simulink model "HDVPSG_DelayComp_NewRef_RealDrop_case1"  (R2019b)
settings: Solver=FixedStepDiscrete  StartTime=0.0  StopTime=28  FixedStep=UT.Ts_Veh  RelTol=1e-3
PostLoadFcn:
  | if any(exist('dsrtsu_mdlpostloadfcn', 'file') ~= 0), dsrtsu_mdlpostloadfcn('Execute', bdroot); end
InitFcn:
  | , if any(exist('dsmpb_private', 'file') ~= 0), dsmpb_private('dsmpb_mdlclblib', 'Init', bdroot); end,
values from neighbouring files (symbols this model uses):
  BETA_HDV_Leader = 50    [HDVPSG_DelayComp_NewRef_RealDrop_script_case1.m]
  BETA_PSG_Follower = 150    [HDVPSG_DelayComp_NewRef_RealDrop_script_case1.m]
  CtrlZone_Length = 250    [HDVPSG_DelayComp_NewRef_RealDrop_script_case1.m]
  DELTA_D_MIN = 5    [HDVPSG_DelayComp_NewRef_RealDrop_script_case1.m]
  DELTA_DR_MG_TCC = 15    [HDVPSG_DelayComp_NewRef_RealDrop_script_case1.m]
  HDV_AMAX = 1.3    [HDVPSG_DelayComp_NewRef_RealDrop_script_case1.m]
  HDV_AMIN = -2.5    [HDVPSG_DelayComp_NewRef_RealDrop_script_case1.m]
  HDV_first_v0 = 13    [HDVPSG_DelayComp_NewRef_RealDrop_script_case1.m]
  HDV_HighMu_D = 9    [HDVPSG_DelayComp_NewRef_RealDrop_script_case1.m]
  HDV_HighMu_I = 27    [HDVPSG_DelayComp_NewRef_RealDrop_script_case1.m]
  HDV_HighMu_P = 27    [HDVPSG_DelayComp_NewRef_RealDrop_script_case1.m]
  HDV_HighMu_TRFC = 0.7    [HDVPSG_DelayComp_NewRef_RealDrop_script_case1.m]
  HDV_last_v0 = 13    [HDVPSG_DelayComp_NewRef_RealDrop_script_case1.m]
  HDV_LowMu_D = 6    [HDVPSG_DelayComp_NewRef_RealDrop_script_case1.m]
  HDV_LowMu_I = 8    [HDVPSG_DelayComp_NewRef_RealDrop_script_case1.m]
  HDV_LowMu_P = 12    [HDVPSG_DelayComp_NewRef_RealDrop_script_case1.m]
  HDV_LowMu_TRFC = 0.6    [HDVPSG_DelayComp_NewRef_RealDrop_script_case1.m]
  Np_MPC = 20    [HDVPSG_DelayComp_NewRef_RealDrop_script_case1.m]
  PSG_AMAX = 3.2    [HDVPSG_DelayComp_NewRef_RealDrop_script_case1.m]
  PSG_AMIN = -6    [HDVPSG_DelayComp_NewRef_RealDrop_script_case1.m]
  PSG_end_v0 = 13    [HDVPSG_DelayComp_NewRef_RealDrop_script_case1.m]
  PSG_first_v0 = 13    [HDVPSG_DelayComp_NewRef_RealDrop_script_case1.m]
  PSG_HighMu_D = 15    [HDVPSG_DelayComp_NewRef_RealDrop_script_case1.m]
  PSG_HighMu_I = 125    [HDVPSG_DelayComp_NewRef_RealDrop_script_case1.m]
  PSG_HighMu_P = 75    [HDVPSG_DelayComp_NewRef_RealDrop_script_case1.m]
  PSG_HighMu_TRFC = 0.8    [HDVPSG_DelayComp_NewRef_RealDrop_script_case1.m]
  PSG_LowMu_D = 12    [HDVPSG_DelayComp_NewRef_RealDrop_script_case1.m]
  PSG_LowMu_I = 64    [HDVPSG_DelayComp_NewRef_RealDrop_script_case1.m]
  PSG_LowMu_P = 48    [HDVPSG_DelayComp_NewRef_RealDrop_script_case1.m]
  PSG_LowMu_TRFC = 0.7    [HDVPSG_DelayComp_NewRef_RealDrop_script_case1.m]
  PSG_middle_v0 = 13    [HDVPSG_DelayComp_NewRef_RealDrop_script_case1.m]
  Q_Leader = 1    [HDVPSG_DelayComp_NewRef_RealDrop_script_case1.m]
  Qd_dot_PSG_Follower = 2    [HDVPSG_DelayComp_NewRef_RealDrop_script_case1.m]
  Qd_PSG_Follower = 10    [HDVPSG_DelayComp_NewRef_RealDrop_script_case1.m]
  R_Leader = 20    [HDVPSG_DelayComp_NewRef_RealDrop_script_case1.m]
  R_PSG_Follower = 1    [HDVPSG_DelayComp_NewRef_RealDrop_script_case1.m]
  Recved_40_1 = Recved_Flag_Combined(47740,:)    [HDVPSG_DelayComp_NewRef_RealDrop_script_case1.m]
  Recved_40_2 = Recved_Flag_Combined(47780,:)    [HDVPSG_DelayComp_NewRef_RealDrop_script_case1.m]
  Recved_40_3 = Recved_Flag_Combined(49536,:)    [HDVPSG_DelayComp_NewRef_RealDrop_script_case1.m]
  Recved_40_4 = Recved_Flag_Combined(118106,:)    [HDVPSG_DelayComp_NewRef_RealDrop_script_case1.m]
  Rho_deltad_PSG_Follower = 1e3    (= 1000)    [HDVPSG_DelayComp_NewRef_RealDrop_script_case1.m]
  Rho_v_PSG_Follower = 1e3    (= 1000)    [HDVPSG_DelayComp_NewRef_RealDrop_script_case1.m]
  T_ADE = 0.01    [HDVPSG_DelayComp_NewRef_RealDrop_script_case1.m]
  V_MAX = 40    [HDVPSG_DelayComp_NewRef_RealDrop_script_case1.m]
  V_MIN = 0    [HDVPSG_DelayComp_NewRef_RealDrop_script_case1.m]
  VR_MG_TCC = 15    [HDVPSG_DelayComp_NewRef_RealDrop_script_case1.m]
undefined symbols (not defined in the file or in its folder): DiscIntNeverNeededParam, UT
libraries: simulink x46
(part 16 of 16)

== matlab function HDVPSG_DelayComp_NewRef_RealDrop_case1/Subsystem6/Subsystem17/MATLAB Function ==
  data: distMP input; HighTRFC output
function HighTRFC = fcn(distMP)
    if distMP<=150 && distMP>=120
        HighTRFC = 0; % iced road 
    else 
        HighTRFC = 1;
    end 
end

== matlab function HDVPSG_DelayComp_NewRef_RealDrop_case1/Subsystem6/Subsystem16/MATLAB Function ==
  data: distMP input; HighTRFC output
function HighTRFC = fcn(distMP)
    if distMP<=150 && distMP>=120
        HighTRFC = 0; % iced road 
    else 
        HighTRFC = 1;
    end 
end

== matlab function HDVPSG_DelayComp_NewRef_RealDrop_case1/Subsystem3/Subsystem17/MATLAB Function ==
  data: distMP input; HighTRFC output
function HighTRFC = fcn(distMP)
    if distMP<=150 && distMP>=120
        HighTRFC = 0; % iced road 
    else 
        HighTRFC = 1;
    end 
end

== matlab function HDVPSG_DelayComp_NewRef_RealDrop_case1/Subsystem3/Subsystem18/MATLAB Function ==
  data: distMP input; HighTRFC output
function HighTRFC = fcn(distMP)
    if distMP<=150 && distMP>=120
        HighTRFC = 0; % iced road 
    else 
        HighTRFC = 1;
    end 
end

== matlab function HDVPSG_DelayComp_NewRef_RealDrop_case1/Subsystem3/Subsystem7/MATLAB Function ==
  data: distMP input; HighTRFC output
function HighTRFC = fcn(distMP)
    if distMP<=150 && distMP>=120
        HighTRFC = 0; % iced road 
    else 
        HighTRFC = 1;
    end 
end

== matlab function HDVPSG_DelayComp_NewRef_RealDrop_case1/Subsystem12/ARE_First_Order_Derivative_[1,0,0]5/MATLAB Function ==
  data: U input; Dot_U output; Ts input; u_init input
function Dot_U = buffer(U, Ts, u_init)
    N = 12
    %Ts = 0.01;
    persistent y;
    if isempty(y)
        y=u_init*ones(N+1,1);%m/s
    end

    y = [U;y(1:end-1)];
    T = Ts*N;
    P = zeros(1,N+1);
    P_alpha = P;
    for k = 1:N+1
        tao_k = (k-1)*Ts;
        P(k) = T-2*tao_k;
        if((k==1)||(k==N+1))
            P_alpha(k) = P(k)*Ts/2;
        else
            P_alpha(k) = P(k)*Ts;
        end
    end
    
    Dot_U = P_alpha*y*6/(T^3);

end

== matlab function HDVPSG_DelayComp_NewRef_RealDrop_case1/PSG1_control_withPDR_compen/Sys3 ==
  data: Ts input; A output; B output; dk output; beta input; delta_d_ddot_hat input
function [A, B, dk] = Sys(Ts, beta, delta_d_ddot_hat)
    A = [1  Ts;
         0  1];
    
    B =  [0; -beta*Ts];
    
    dk = [0; delta_d_ddot_hat*Ts];
end

== matlab function HDVPSG_DelayComp_NewRef_RealDrop_case1/HDV2_control_withPDR_compen/Subsystem17/Poly_coefficient ==
  data: a_0 output; delta_d0 input; a_1 output; a_2 output; delta_dTCC input; delta_v0 input; Tend input; a_3 output
function [a_0, a_1, a_2, a_3] = poly_4_coefficient(delta_d0, delta_dTCC, delta_v0, Tend)
% With conditions:
% delta_d_0 given,            delta_v_0 given 
% delta_d_Tend = delta_d_TTC, delta_v_Tend = 0

% delta_dr(t) = a0 + a1*t + a2*t^2 + a3*t^3
    a_0 = delta_d0;
    a_1 = delta_v0;
    a_2 = -(3*delta_d0 - 3*delta_dTCC + 2*Tend*delta_v0)/Tend^2;
    a_3 = (2*delta_d0 - 2*delta_dTCC + Tend*delta_v0)/Tend^3;
end

== matlab function HDVPSG_DelayComp_NewRef_RealDrop_case1/HDV2_control_withPDR_compen/Subsystem18/Ref ==
  data: delta_dr output; a_0 input; delta_dr_dot output; a_1 input; a_2 input; a_3 input; t_sumo input
function [delta_dr, delta_dr_dot] = poly_4_reference(a_0, a_1, a_2, a_3, t_sumo)
    delta_dr     = a_0 + a_1*t_sumo + a_2*t_sumo^2 + a_3*t_sumo^3;
    delta_dr_dot =       a_1        + 2*a_2*t_sumo + 3*a_3*t_sumo^2;
end

== matlab function HDVPSG_DelayComp_NewRef_RealDrop_case1/HDV2_control_withPDR_compen/Subsystem18/Ref_Pre_Vec ==
  data: delta_dr_Pre_Vec output; a_0 input; delta_dr_dot_Pre_Vec output; a_1 input; a_2 input; a_3 input; t_sumo input
function [delta_dr_Pre_Vec, delta_dr_dot_Pre_Vec] = poly_4_reference(a_0, a_1, a_2, a_3, t_sumo)
    Ts = 0.01;
    Np = 20;
    
    t_Pre_Vec = t_sumo + (1:Np+1)*Ts;
    
    delta_dr_Pre_Vec     = a_0 + a_1*t_Pre_Vec + a_2*t_Pre_Vec.^2 + a_3*t_Pre_Vec.^3;
    delta_dr_dot_Pre_Vec =       a_1           + 2*a_2*t_Pre_Vec  + 3*a_3*t_Pre_Vec.^2;
end

== matlab function HDVPSG_DelayComp_NewRef_RealDrop_case1/HDV2_control_withPDR_compen/Sys3 ==
  data: Ts input; A output; B output; dk output; beta input; delta_d_ddot_hat input
function [A, B, dk] = Sys(Ts, beta, delta_d_ddot_hat)
    A = [1  Ts;
         0  1];
    
    B =  [0; -beta*Ts];
    
    dk = [0; delta_d_ddot_hat*Ts];
end
